simulink model "stepperMotorADRCFirstOrder_originalModel"  (R2026a)
settings: Solver=FixedStepDiscrete  StopTime=1  FixedStep=1e-7
undefined symbols (not defined in the file): alpha_iqd, alpha_s, beta_iqd, beta_s, biq, bs, convert_adc_to_integer, DiscIntNeverNeededParam, electricalRadiansPerCount, gam_iqd, gam_s, k1_iqd, k1_s, KPth, mechanicalRadiansPerCount, PWMVoltage, theta_ref, vs
libraries: simulink x2, mcbeeMathTransformLib x2
settings Model: Creator=mike  LastModifiedBy=drew
settings OptimizationCC: ConditionallyExecuteInputs=off
settings HardwareCC: ProdHWDeviceType=ASIC/FPGA->ASIC/FPGA  TargetBitPerLong=64.0  TargetBitPerPointer=64.0  TargetBitPerSizeT=64.0  TargetBitPerPtrDiffT=64.0  TargetLongLongMode=on  TargetIntDivRoundTo=Zero  TargetEndianess=LittleEndian  TargetWordSize=64.0  TargetHWDeviceType=Custom Processor->MATLAB Host Computer  ProdEqTarget=off

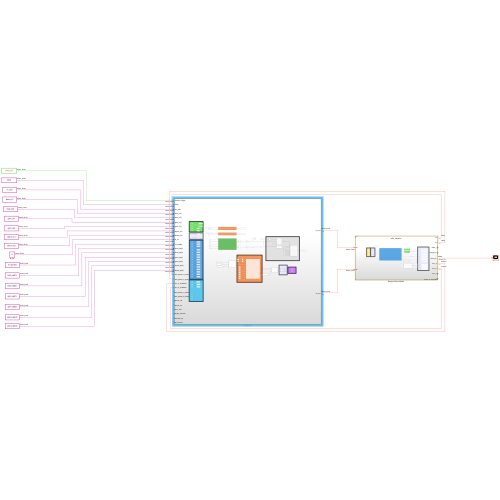
[thumbnail: Simulink's stored preview of the top-level diagram]
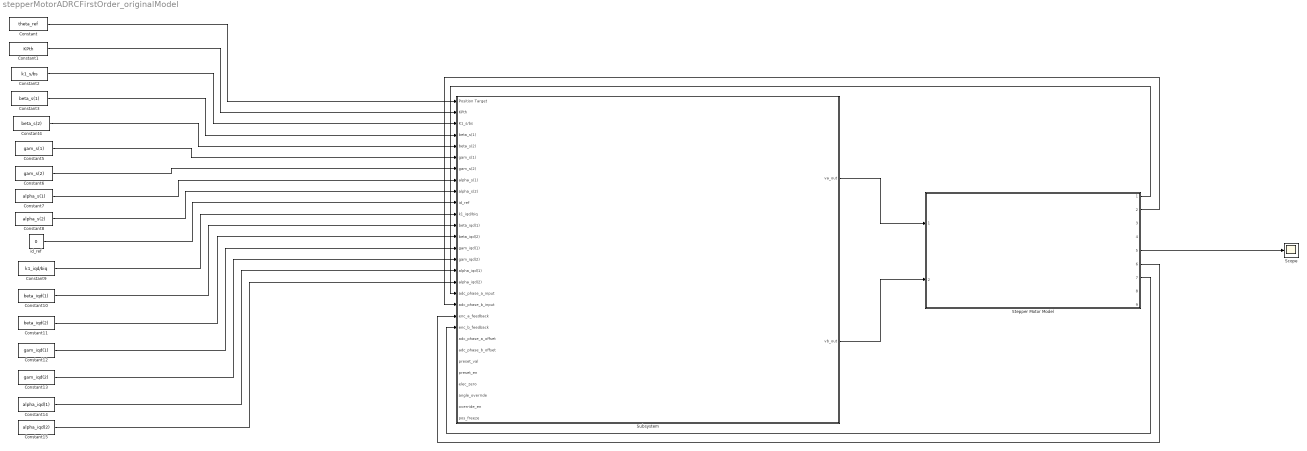
== system stepperMotorADRCFirstOrder_originalModel ==
  Constant : Constant  Value=theta_ref  OutDataTypeStr=PosType  SampleTime=-1
  Constant1 : Constant  Value=KPth  OutDataTypeStr=ParamType
  Constant10 : Constant  Value=beta_iqd(1)  OutDataTypeStr=ParamType
  Constant11 : Constant  Value=beta_iqd(2)  OutDataTypeStr=ParamType
  Constant12 : Constant  Value=gam_iqd(1)  OutDataTypeStr=ParamType
  Constant13 : Constant  Value=gam_iqd(2)  OutDataTypeStr=ParamType
  Constant14 : Constant  Value=alpha_iqd(1)  OutDataTypeStr=ParamType
  Constant15 : Constant  Value=alpha_iqd(2)  OutDataTypeStr=ParamType
  Constant2 : Constant  Value=k1_s/bs  OutDataTypeStr=ParamType
  Constant3 : Constant  Value=beta_s(1)  OutDataTypeStr=ParamType
  Constant4 : Constant  Value=beta_s(2)  OutDataTypeStr=ParamType
  Constant5 : Constant  Value=gam_s(1)  OutDataTypeStr=ParamType
  Constant6 : Constant  Value=gam_s(2)  OutDataTypeStr=ParamType
  Constant7 : Constant  Value=alpha_s(1)  OutDataTypeStr=ParamType
  Constant8 : Constant  Value=alpha_s(2)  OutDataTypeStr=ParamType
  Constant9 : Constant  Value=k1_iqd/biq  OutDataTypeStr=ParamType
  Scope : Scope
      settings: ActiveDisplayYMinimum=-2.1882188276409535  ActiveDisplayYMaximum=0.47029043106523327
  "Stepper Motor Model " : Subsystem  ReferencedSubsystem=adrc_harness
  Subsystem : Subsystem
  id_ref : Constant  Value=0  OutDataTypeStr=ParamType
  wires:
  Constant/1 -> Subsystem/1(Position Target)
  Constant1/1 -> Subsystem/2(KPth)
  Constant2/1 -> Subsystem/3(K1_s/bs)
  Constant3/1 -> Subsystem/4(beta_s(1))
  Constant4/1 -> Subsystem/5(beta_s(2))
  Constant5/1 -> Subsystem/6(gam_s(1))
  Constant6/1 -> Subsystem/7(gam_s(2))
  Constant7/1 -> Subsystem/8(alpha_s(1))
  Constant8/1 -> Subsystem/9(alpha_s(2))
  id_ref/1 -> Subsystem/10(id_ref)
  Constant9/1 -> Subsystem/11(k1_iqd/biq)
  Constant10/1 -> Subsystem/12(beta_iqd(1))
  Constant11/1 -> Subsystem/13(beta_iqd(2))
  Constant12/1 -> Subsystem/14(gam_iqd(1))
  Constant13/1 -> Subsystem/15(gam_iqd(2))
  Constant14/1 -> Subsystem/16(alpha_iqd(1))
  Constant15/1 -> Subsystem/17(alpha_iqd(2))
  Subsystem/1(va_out) -> "Stepper Motor Model "/1
  Subsystem/2(vb_out) -> "Stepper Motor Model "/2
  "Stepper Motor Model "/7 -> Subsystem/21(enc_b_feedback)
  "Stepper Motor Model "/6 -> Subsystem/20(enc_a_feedback)
  "Stepper Motor Model "/1 -> Subsystem/18(adc_phase_a_input)
  "Stepper Motor Model "/2 -> Subsystem/19(adc_phase_b_input)
  "Stepper Motor Model "/5 -> Scope/1

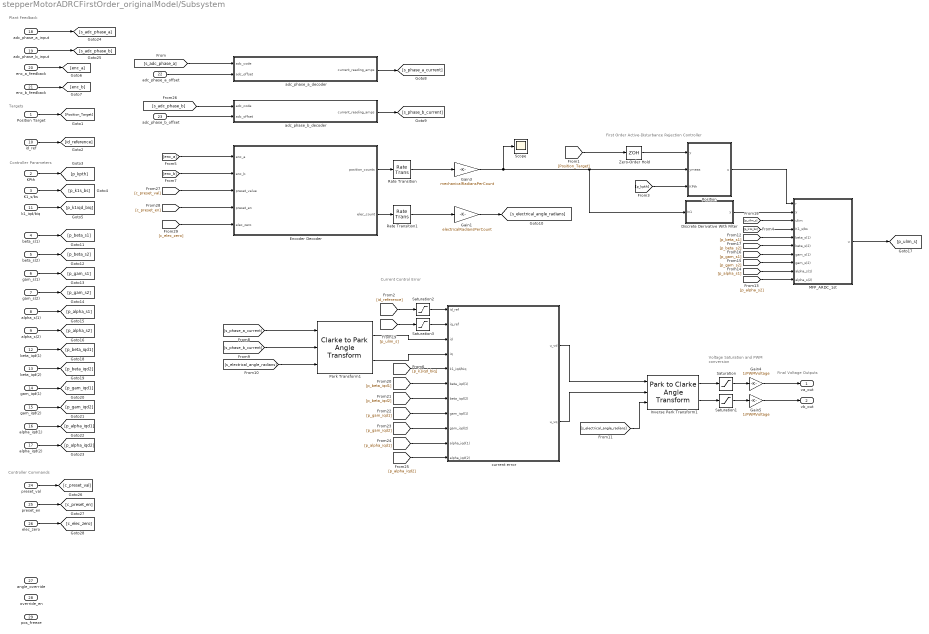
== system stepperMotorADRCFirstOrder_originalModel/Subsystem ==
  note: Final Voltage Outputs
  note: Voltage Saturation and
      | PWM conversion
  note: Current Control Error
  note: First Order Active-Disturbance Rejection Controller
  note: Controller Commands
  note: Controller Parameters
  note: Targets
  note: Plant Feedback
  Position Target : Inport  OutDataTypeStr=PosType
  KPth : Inport  Port=2  OutDataTypeStr=ParamType
  K1_s/bs : Inport  Port=3  OutDataTypeStr=ParamType
  beta_s(1) : Inport  Port=4  OutDataTypeStr=ParamType
  beta_s(2) : Inport  Port=5  OutDataTypeStr=ParamType
  gam_s(1) : Inport  Port=6  OutDataTypeStr=ParamType
  gam_s(2) : Inport  Port=7  OutDataTypeStr=ParamType
  alpha_s(1) : Inport  Port=8  OutDataTypeStr=ParamType
  alpha_s(2) : Inport  Port=9  OutDataTypeStr=ParamType
  id_ref : Inport  Port=10  OutDataTypeStr=ParamType
  k1_iqd/biq : Inport  Port=11  OutDataTypeStr=ParamType
  beta_iqd(1) : Inport  Port=12  OutDataTypeStr=ParamType
  beta_iqd(2) : Inport  Port=13  OutDataTypeStr=ParamType
  gam_iqd(1) : Inport  Port=14  OutDataTypeStr=ParamType
  gam_iqd(2) : Inport  Port=15  OutDataTypeStr=ParamType
  alpha_iqd(1) : Inport  Port=16  OutDataTypeStr=ParamType
  alpha_iqd(2) : Inport  Port=17  OutDataTypeStr=ParamType
  adc_phase_a_input : Inport  Port=18
  adc_phase_b_input : Inport  Port=19
  enc_a_feedback : Inport  Port=20
  enc_b_feedback : Inport  Port=21
  adc_phase_a_offset : Inport  Port=22  OutDataTypeStr=uint16
  adc_phase_b_offset : Inport  Port=23  OutDataTypeStr=uint16
  preset_val : Inport  Port=24  OutDataTypeStr=fixdt(1,32,0)
  preset_en : Inport  Port=25  OutDataTypeStr=boolean
  elec_zero : Inport  Port=26  OutDataTypeStr=boolean
  angle_override : Inport  Port=27  OutDataTypeStr=uint16
  override_en : Inport  Port=28  OutDataTypeStr=boolean
  pos_freeze : Inport  Port=29  OutDataTypeStr=boolean
  Discrete Derivative With Filter : Subsystem
  Encoder Decoder : Subsystem
  Gain1 : Gain  Gain=electricalRadiansPerCount  OutDataTypeStr=PosType  SaturateOnIntegerOverflow=on
  Gain3 : Gain  Gain=mechanicalRadiansPerCount  OutDataTypeStr=PosType  SaturateOnIntegerOverflow=on
  Gain4 : Gain  Gain=1/PWMVoltage  OutDataTypeStr=ParamType
  Gain5 : Gain  Gain=1/PWMVoltage  OutDataTypeStr=ParamType
  Inverse Park Transform1 : mcbeeMathTransformLib/Park to Clarke Angle Transform  AxisAlignment=D-axis  UseWithEmbedded=on  PhaseInput=Two inputs  ThetaInput=Electrical position  AngleInput=Radians  N_points=1024
      settings: LibrarySourceBlock=mcbhdllib/Controls/Math Transforms/Inverse Park Transform
  MFP_ARDC_1st : Subsystem
  Park Transform1 : mcbeeMathTransformLib/Clarke to Park Angle Transform  AxisAlignment=D-axis  UseWithEmbedded=on  PhaseInput=Two inputs  ThetaInput=Electrical position  AngleInput=Radians  N_points=1024
      settings: LibrarySourceBlock=mcbhdllib/Controls/Math Transforms/Park Transform
  "Position " : Subsystem
  Rate Transition : RateTransition  OutPortSampleTime=2e-5
  Rate Transition1 : RateTransition  OutPortSampleTime=2e-5
  Saturation : Saturate  UpperLimit=PWMVoltage  LowerLimit=-PWMVoltage
  Saturation1 : Saturate  UpperLimit=PWMVoltage  LowerLimit=-PWMVoltage  OutDataTypeStr=ParamType
  Saturation2 : Saturate  UpperLimit=2.4  LowerLimit=-2.4  OutDataTypeStr=ParamType
  Saturation3 : Saturate  UpperLimit=2.4  LowerLimit=-2.4  OutDataTypeStr=ParamType
  Scope : Scope
      settings: DataLoggingVariableName=ScopeData3
  Zero-Order Hold : ZeroOrderHold  SampleTime=2e-5
  adc_phase_a_decoder : Subsystem
  adc_phase_b_decoder : Subsystem
  current error : Subsystem
  va_out : Outport  OutDataTypeStr=ParamType
  vb_out : Outport  Port=2  OutDataTypeStr=ParamType
  wires:
  Inverse Park Transform1/2 -> Saturation1/1
  current error/1(u_vd) -> Inverse Park Transform1/1
  current error/2(u_vq) -> Inverse Park Transform1/2
  Zero-Order Hold/1 -> "Position "/1(y)
  Park Transform1/2 -> current error/4(iq)
  Inverse Park Transform1/1 -> Saturation/1
  Park Transform1/1 -> current error/3(id)
  "Position "/1(u) -> MFP_ARDC_1st/1(r)
  Discrete Derivative With Filter/1(y) -> MFP_ARDC_1st/2(y)
  Saturation/1 -> Gain4/1
  Saturation1/1 -> Gain5/1
  Gain4/1 -> va_out/1
  Gain5/1 -> vb_out/1
  [Position_Target] -> Zero-Order Hold/1
  Position Target/1 -> [Position_Target]
  id_ref/1 -> [id_reference]
  [p_kpth] -> "Position "/3(KPth)
  KPth/1 -> [p_kpth]
  [p_k1s_bs] -> MFP_ARDC_1st/4(K1_s/bs)
  K1_s/bs/1 -> [p_k1s_bs]
  [p_k1iqd_biq] -> current error/5(k1_iqd/biq)
  k1_iqd/biq/1 -> [p_k1iqd_biq]
  adc_phase_a_offset/1 -> adc_phase_a_decoder/2(adc_offset)
  adc_phase_b_offset/1 -> adc_phase_b_decoder/2(adc_offset)
  enc_a_feedback/1 -> [enc_a]
  enc_b_feedback/1 -> [enc_b]
  [enc_a] -> Encoder Decoder/1(enc_a)
  [enc_b] -> Encoder Decoder/2(enc_b)
  adc_phase_a_decoder/1(current_reading_amps) -> [s_phase_a_current]
  adc_phase_b_decoder/1(current_reading_amps) -> [s_phase_b_current]
  [s_phase_a_current] -> Park Transform1/1
  [s_phase_b_current] -> Park Transform1/2
  [s_electrical_angle_radians] -> Park Transform1/3
  [s_electrical_angle_radians] -> Inverse Park Transform1/3
  [p_beta_s1] -> MFP_ARDC_1st/5(beta_s(1))
  [p_beta_s2] -> MFP_ARDC_1st/6(beta_s(2))
  [p_gam_s1] -> MFP_ARDC_1st/7(gam_s(1))
  [p_gam_s2] -> MFP_ARDC_1st/8(gam_s(2))
  [p_alpha_s1] -> MFP_ARDC_1st/9(alpha_s(1))
  [p_alpha_s2] -> MFP_ARDC_1st/10(alpha_s(2))
  alpha_s(2)/1 -> [p_alpha_s2]
  alpha_s(1)/1 -> [p_alpha_s1]
  gam_s(2)/1 -> [p_gam_s2]
  gam_s(1)/1 -> [p_gam_s1]
  beta_s(2)/1 -> [p_beta_s2]
  beta_s(1)/1 -> [p_beta_s1]
  MFP_ARDC_1st/1(u) -> [p_ulim_s]
  [p_ulim_s] -> MFP_ARDC_1st/3(ulim)
  beta_iqd(1)/1 -> [p_beta_iqd1]
  beta_iqd(2)/1 -> [p_beta_iqd2]
  [p_beta_iqd2] -> current error/7(beta_iqd(2))
  [p_beta_iqd1] -> current error/6(beta_iqd(1))
  gam_iqd(2)/1 -> [p_gam_iqd2]
  gam_iqd(1)/1 -> [p_gam_iqd1]
  [p_gam_iqd1] -> current error/8(gam_iqd(1))
  [p_gam_iqd2] -> current error/9(gam_iqd(2))
  [p_alpha_iqd1] -> current error/10(alpha_iqd(1))
  [p_alpha_iqd2] -> current error/11(alpha_iqd(2))
  alpha_iqd(1)/1 -> [p_alpha_iqd1]
  alpha_iqd(2)/1 -> [p_alpha_iqd2]
  adc_phase_a_input/1 -> [s_adc_phase_a]
  adc_phase_b_input/1 -> [s_adc_phase_b]
  [s_adc_phase_a] -> adc_phase_a_decoder/1(adc_code)
  [s_adc_phase_b] -> adc_phase_b_decoder/1(adc_code)
  [c_elec_zero] -> Encoder Decoder/5(elec_zero)
  [c_preset_en] -> Encoder Decoder/4(preset_en)
  [c_preset_val] -> Encoder Decoder/3(preset_value)
  elec_zero/1 -> [c_elec_zero]
  preset_en/1 -> [c_preset_en]
  preset_val/1 -> [c_preset_val]
  [id_reference] -> Saturation2/1
  Saturation2/1 -> current error/1(id_ref)
  [p_ulim_s] -> Saturation3/1
  Saturation3/1 -> current error/2(iq_ref)
  Encoder Decoder/2(elec_count) -> Rate Transition1/1
  Encoder Decoder/1(position_counts) -> Rate Transition/1
  Rate Transition/1 -> Gain3/1
  Rate Transition1/1 -> Gain1/1
  Gain1/1 -> [s_electrical_angle_radians]
  Gain3/1 -> Scope/1, Discrete Derivative With Filter/1(In1), "Position "/2(ymeas)

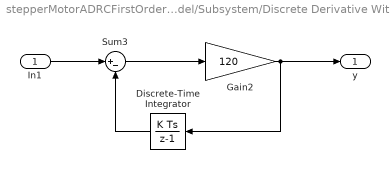
== system stepperMotorADRCFirstOrder_originalModel/Subsystem/Discrete Derivative With Filter ==
  In1 : Inport  OutDataTypeStr=PosType
  Discrete-Time Integrator : DiscreteIntegrator  SampleTime=2e-5  OutDataTypeStr=PosType  SaturateOnIntegerOverflow=on  ICPrevOutput=DiscIntNeverNeededParam  ICPrevScaledInput=DiscIntNeverNeededParam
  Gain2 : Gain  Gain=120  OutDataTypeStr=PosType  ParamDataTypeStr=Inherit: Same as input
  Sum3 : Sum  Inputs=|+-  OutDataTypeStr=PosType
  y : Outport  OutDataTypeStr=PosType
  wires:
  Gain2/1 -> y/1, Discrete-Time Integrator/1
  Sum3/1 -> Gain2/1
  Discrete-Time Integrator/1 -> Sum3/2
  In1/1 -> Sum3/1

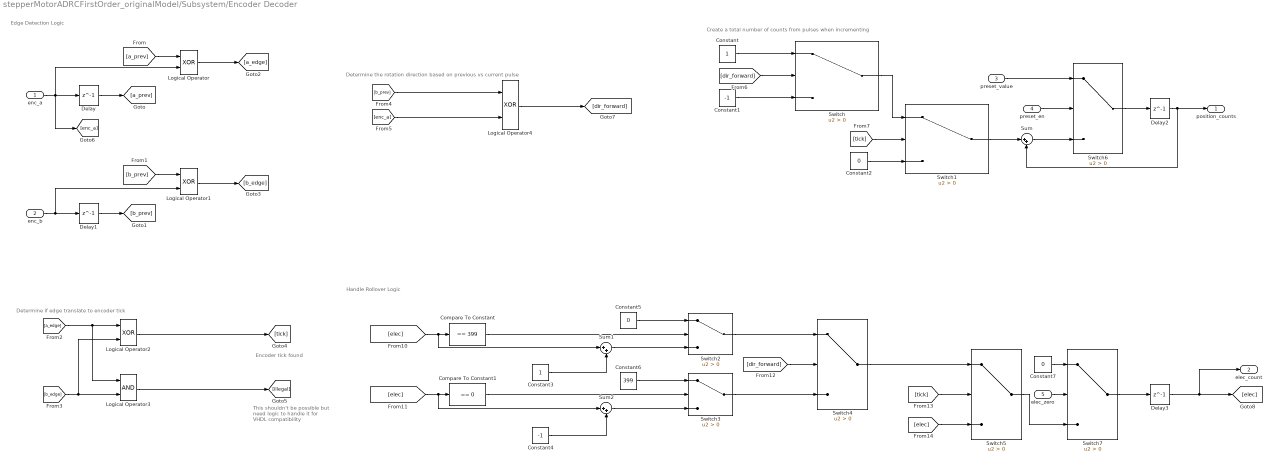
== system stepperMotorADRCFirstOrder_originalModel/Subsystem/Encoder Decoder ==
  note: Handle Rollover Logic
  note: Create a total number of counts from pulses when incrementing
  note: Determine the rotation direction based on previous vs current pulse
  note: Encoder tick found
  note: Determine if edge translate to encoder tick
  note: Edge Detection Logic
  note: This shouldn't be possible but need logic to handle it for VHDL compatibility
  enc_a : Inport  OutDataTypeStr=boolean
  enc_b : Inport  Port=2  OutDataTypeStr=boolean
  preset_value : Inport  Port=3  OutDataTypeStr=fixdt(1,32,0)
  preset_en : Inport  Port=4  OutDataTypeStr=boolean
  elec_zero : Inport  Port=5  OutDataTypeStr=boolean
  Compare To Constant : simulink/Logic and Bit Operations/Compare To Constant  relop===  const=399  OutDataTypeStr=boolean
  Compare To Constant1 : simulink/Logic and Bit Operations/Compare To Constant  relop===  const=0  OutDataTypeStr=boolean
  Constant : Constant  OutDataTypeStr=int32
  Constant1 : Constant  Value=-1  OutDataTypeStr=int32
  Constant2 : Constant  Value=0  OutDataTypeStr=int32
  Constant3 : Constant  OutDataTypeStr=int32
  Constant4 : Constant  Value=-1  OutDataTypeStr=int32
  Constant5 : Constant  Value=0  OutDataTypeStr=int32
  Constant6 : Constant  Value=399  OutDataTypeStr=int32
  Constant7 : Constant  Value=0  OutDataTypeStr=int32
  Delay{,1..3} (4 alike) : Delay  DelayLength=1  InputProcessing=Columns as channels (frame based)  SampleTime=1e-7
  Logical Operator{,1..2,4} (4 alike) : Logic  Operator=XOR  AllPortsSameDT=off  OutDataTypeStr=boolean
  Logical Operator3 : Logic  AllPortsSameDT=off  OutDataTypeStr=boolean
  Sum : Sum  Inputs=|++  OutDataTypeStr=int32  SaturateOnIntegerOverflow=on
  Sum1 : Sum  Inputs=|++  OutDataTypeStr=int32
  Sum2 : Sum  Inputs=|++  OutDataTypeStr=int32
  Switch{,1..5} (6 alike) : Switch  Criteria=u2 > Threshold  SaturateOnIntegerOverflow=off  InputSameDT=off
  Switch6 : Switch  Criteria=u2 > Threshold  OutDataTypeStr=CountType  SaturateOnIntegerOverflow=off  InputSameDT=off
  Switch7 : Switch  Criteria=u2 > Threshold  OutDataTypeStr=CountType  SaturateOnIntegerOverflow=off  InputSameDT=off
  position_counts : Outport  OutDataTypeStr=CountType
  elec_count : Outport  Port=2  OutDataTypeStr=CountType
  wires:
  enc_b/1 -> Logical Operator1/2, Delay1/1
  enc_a/1 -> [enc_a], Logical Operator/2, Delay/1
  Delay/1 -> [a_prev]
  Delay1/1 -> [b_prev]
  [b_prev] -> Logical Operator1/1
  [a_prev] -> Logical Operator/1
  Logical Operator/1 -> [a_edge]
  Logical Operator1/1 -> [b_edge]
  [b_edge] -> Logical Operator3/2, Logical Operator2/2
  [a_edge] -> Logical Operator2/1, Logical Operator3/1
  Logical Operator2/1 -> [tick]
  Logical Operator3/1 -> [illegal]
  [b_prev] -> Logical Operator4/1
  [enc_a] -> Logical Operator4/2
  Logical Operator4/1 -> [dir_forward]
  Constant/1 -> Switch/1
  Constant1/1 -> Switch/3
  [dir_forward] -> Switch/2
  [tick] -> Switch1/2
  Constant2/1 -> Switch1/3
  Switch/1 -> Switch1/1
  Switch1/1 -> Sum/1
  Delay2/1 -> position_counts/1, Sum/2
  Constant5/1 -> Switch2/1
  Compare To Constant1/1 -> Switch3/2
  Sum2/1 -> Switch3/3
  Sum1/1 -> Switch2/3
  Constant6/1 -> Switch3/1
  [elec] -> Sum2/1, Compare To Constant1/1
  [elec] -> Sum1/1, Compare To Constant/1
  Switch2/1 -> Switch4/1
  Constant3/1 -> Sum1/2
  Compare To Constant/1 -> Switch2/2
  Constant4/1 -> Sum2/2
  [dir_forward] -> Switch4/2
  Switch3/1 -> Switch4/3
  Switch4/1 -> Switch5/1
  [tick] -> Switch5/2
  [elec] -> Switch5/3
  Delay3/1 -> elec_count/1, [elec]
  Sum/1 -> Switch6/3
  Switch6/1 -> Delay2/1
  preset_en/1 -> Switch6/2
  preset_value/1 -> Switch6/1
  Constant7/1 -> Switch7/1
  elec_zero/1 -> Switch7/2
  Switch5/1 -> Switch7/3
  Switch7/1 -> Delay3/1

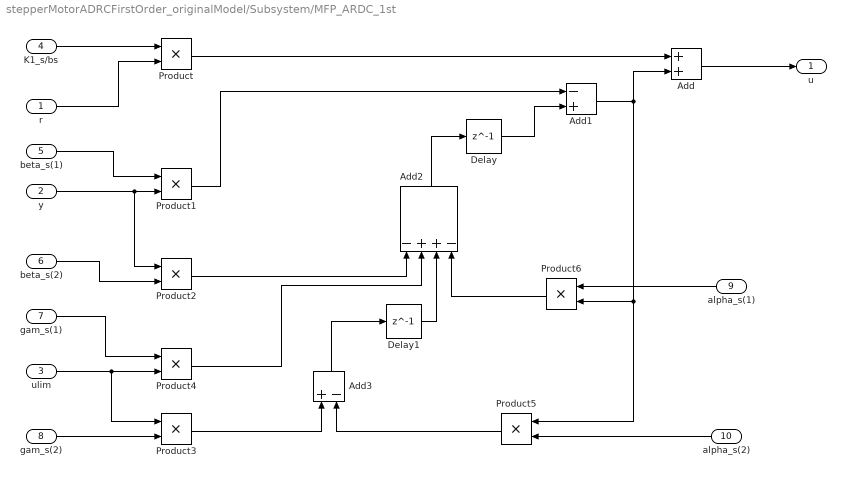
== system stepperMotorADRCFirstOrder_originalModel/Subsystem/MFP_ARDC_1st ==
  r : Inport  OutDataTypeStr=PosType
  y : Inport  Port=2  OutDataTypeStr=PosType
  ulim : Inport  Port=3  OutDataTypeStr=ParamType
  K1_s/bs : Inport  Port=4  OutDataTypeStr=ParamType
  beta_s(1) : Inport  Port=5  OutDataTypeStr=ParamType
  beta_s(2) : Inport  Port=6  OutDataTypeStr=ParamType
  gam_s(1) : Inport  Port=7  OutDataTypeStr=ParamType
  gam_s(2) : Inport  Port=8  OutDataTypeStr=ParamType
  alpha_s(1) : Inport  Port=9  OutDataTypeStr=ParamType
  alpha_s(2) : Inport  Port=10  OutDataTypeStr=ParamType
  Add : Sum  OutDataTypeStr=ParamType  SaturateOnIntegerOverflow=on
  Add1 : Sum  Inputs=-+  OutDataTypeStr=ParamType  SaturateOnIntegerOverflow=on
  Add2 : Sum  Inputs=-++-  OutDataTypeStr=ParamType  SaturateOnIntegerOverflow=on
  Add3 : Sum  Inputs=+-  OutDataTypeStr=ParamType  SaturateOnIntegerOverflow=on
  Delay : Delay  DelayLength=1  InitialCondition=0  SampleTime=2e-5
  Delay1 : Delay  DelayLength=1  InitialCondition=0  SampleTime=2e-5
  Product{,1..6} (7 alike) : Product  OutDataTypeStr=ParamType  SaturateOnIntegerOverflow=on
  u : Outport  OutDataTypeStr=ParamType
  wires:
  Add/1 -> u/1
  Add3/1 -> Delay1/1
  Product4/1 -> Add2/2
  Product6/1 -> Add2/4
  Add1/1 -> Product5/1, Product6/2, Add/2
  Add2/1 -> Delay/1
  r/1 -> Product/2
  Delay1/1 -> Add2/3
  Product3/1 -> Add3/1
  ulim/1 -> Product3/1, Product4/2
  Product2/1 -> Add2/1
  Product5/1 -> Add3/2
  Delay/1 -> Add1/2
  Product1/1 -> Add1/1
  y/1 -> Product2/1, Product1/2
  K1_s/bs/1 -> Product/1
  Product/1 -> Add/1
  beta_s(1)/1 -> Product1/1
  beta_s(2)/1 -> Product2/2
  gam_s(1)/1 -> Product4/1
  gam_s(2)/1 -> Product3/2
  alpha_s(2)/1 -> Product5/2
  alpha_s(1)/1 -> Product6/1

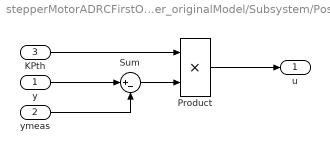
== system stepperMotorADRCFirstOrder_originalModel/Subsystem/Position  ==
  y : Inport  OutDataTypeStr=PosType
  ymeas : Inport  Port=2  OutDataTypeStr=PosType
  KPth : Inport  Port=3  OutDataTypeStr=ParamType
  Product : Product  OutDataTypeStr=PosType  SaturateOnIntegerOverflow=on
  Sum : Sum  Inputs=|+-  OutDataTypeStr=PosType  SaturateOnIntegerOverflow=on
  u : Outport  OutDataTypeStr=PosType
  wires:
  y/1 -> Sum/1
  ymeas/1 -> Sum/2
  Sum/1 -> Product/2
  Product/1 -> u/1
  KPth/1 -> Product/1

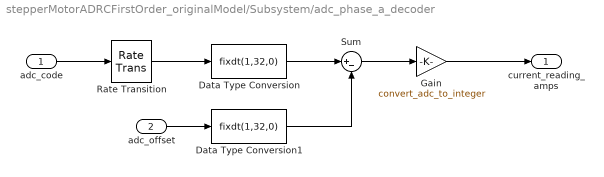
== system stepperMotorADRCFirstOrder_originalModel/Subsystem/adc_phase_a_decoder ==
  adc_code : Inport  OutMin=[0]  OutDataTypeStr=uint16
  adc_offset : Inport  Port=2  OutDataTypeStr=uint16
  Data Type Conversion : DataTypeConversion  OutDataTypeStr=fixdt(1,32,0)  RndMeth=Floor
  Data Type Conversion1 : DataTypeConversion  OutDataTypeStr=fixdt(1,32,0)  RndMeth=Floor
  Gain : Gain  Gain=convert_adc_to_integer  ParamDataTypeStr=fixdt(0,32,38)  OutDataTypeStr=ParamType  RndMeth=Nearest  SaturateOnIntegerOverflow=on
  Rate Transition : RateTransition  OutPortSampleTime=2e-5
  Sum : Sum  Inputs=|+-  OutDataTypeStr=ParamType  AccumDataTypeStr=fixdt(1,32,0)  SaturateOnIntegerOverflow=on
  current_reading_amps : Outport  OutDataTypeStr=ParamType
  wires:
  adc_offset/1 -> Data Type Conversion1/1
  Data Type Conversion1/1 -> Sum/2
  Data Type Conversion/1 -> Sum/1
  Sum/1 -> Gain/1
  Gain/1 -> current_reading_amps/1
  adc_code/1 -> Rate Transition/1
  Rate Transition/1 -> Data Type Conversion/1

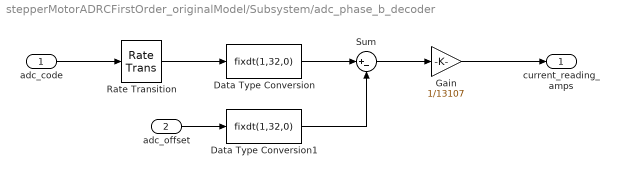
== system stepperMotorADRCFirstOrder_originalModel/Subsystem/adc_phase_b_decoder ==
  adc_code : Inport  OutMin=[0]  OutDataTypeStr=uint16
  adc_offset : Inport  Port=2  OutDataTypeStr=uint16
  Data Type Conversion : DataTypeConversion  OutDataTypeStr=fixdt(1,32,0)  RndMeth=Floor
  Data Type Conversion1 : DataTypeConversion  OutDataTypeStr=fixdt(1,32,0)  RndMeth=Floor
  Gain : Gain  Gain=1/13107  ParamDataTypeStr=fixdt(0,32,38)  OutDataTypeStr=ParamType  RndMeth=Nearest  SaturateOnIntegerOverflow=on
  Rate Transition : RateTransition  OutPortSampleTime=2e-5
  Sum : Sum  Inputs=|+-  OutDataTypeStr=ParamType  AccumDataTypeStr=fixdt(1,32,0)  SaturateOnIntegerOverflow=on
  current_reading_amps : Outport  OutDataTypeStr=ParamType
  wires:
  adc_offset/1 -> Data Type Conversion1/1
  Data Type Conversion1/1 -> Sum/2
  Data Type Conversion/1 -> Sum/1
  Sum/1 -> Gain/1
  Gain/1 -> current_reading_amps/1
  Rate Transition/1 -> Data Type Conversion/1
  adc_code/1 -> Rate Transition/1

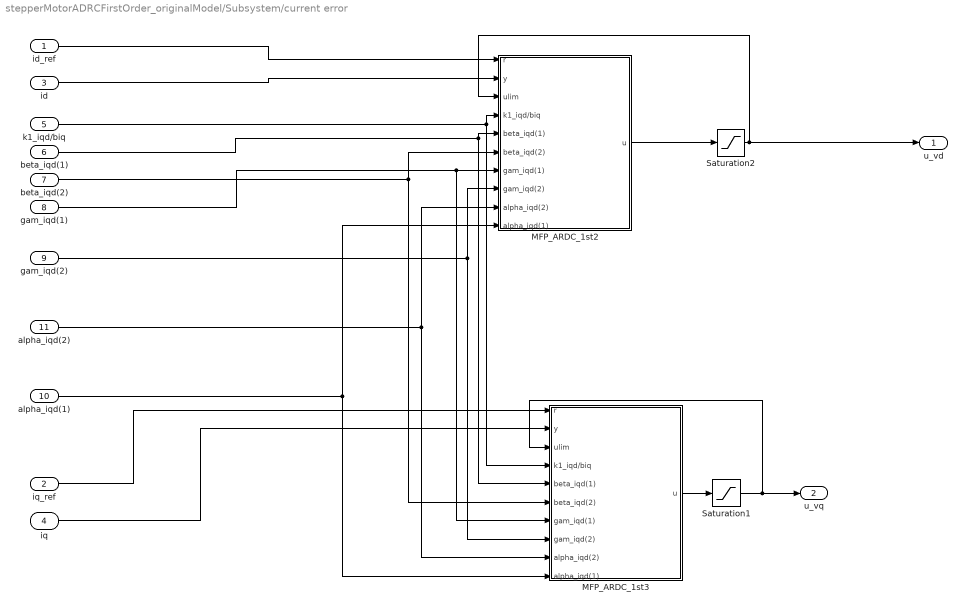
== system stepperMotorADRCFirstOrder_originalModel/Subsystem/current error ==
  id_ref : Inport  OutDataTypeStr=ParamType
  iq_ref : Inport  Port=2  OutDataTypeStr=ParamType
  id : Inport  Port=3  OutDataTypeStr=ParamType
  iq : Inport  Port=4  OutDataTypeStr=ParamType
  k1_iqd/biq : Inport  Port=5  OutDataTypeStr=ParamType
  beta_iqd(1) : Inport  Port=6  OutDataTypeStr=ParamType
  beta_iqd(2) : Inport  Port=7  OutDataTypeStr=ParamType
  gam_iqd(1) : Inport  Port=8  OutDataTypeStr=ParamType
  gam_iqd(2) : Inport  Port=9  OutDataTypeStr=ParamType
  alpha_iqd(1) : Inport  Port=10  OutDataTypeStr=ParamType
  alpha_iqd(2) : Inport  Port=11  OutDataTypeStr=ParamType
  MFP_ARDC_1st2 : Subsystem
  MFP_ARDC_1st3 : Subsystem
  Saturation1 : Saturate  UpperLimit=vs  LowerLimit=-vs  OutDataTypeStr=ParamType
  Saturation2 : Saturate  UpperLimit=vs  LowerLimit=-vs  OutDataTypeStr=ParamType
  u_vd : Outport  OutDataTypeStr=ParamType
  u_vq : Outport  Port=2  OutDataTypeStr=ParamType
  wires:
  iq_ref/1 -> MFP_ARDC_1st3/1(r)
  iq/1 -> MFP_ARDC_1st3/2(y)
  Saturation1/1 -> MFP_ARDC_1st3/3(ulim), u_vq/1
  MFP_ARDC_1st3/1(u) -> Saturation1/1
  id/1 -> MFP_ARDC_1st2/2(y)
  id_ref/1 -> MFP_ARDC_1st2/1(r)
  MFP_ARDC_1st2/1(u) -> Saturation2/1
  Saturation2/1 -> MFP_ARDC_1st2/3(ulim), u_vd/1
  k1_iqd/biq/1 -> MFP_ARDC_1st2/4(k1_iqd/biq), MFP_ARDC_1st3/4(k1_iqd/biq)
  beta_iqd(1)/1 -> MFP_ARDC_1st2/5(beta_iqd(1)), MFP_ARDC_1st3/5(beta_iqd(1))
  beta_iqd(2)/1 -> MFP_ARDC_1st3/6(beta_iqd(2)), MFP_ARDC_1st2/6(beta_iqd(2))
  gam_iqd(1)/1 -> MFP_ARDC_1st2/7(gam_iqd(1)), MFP_ARDC_1st3/7(gam_iqd(1))
  gam_iqd(2)/1 -> MFP_ARDC_1st2/8(gam_iqd(2)), MFP_ARDC_1st3/8(gam_iqd(2))
  alpha_iqd(2)/1 -> MFP_ARDC_1st2/9(alpha_iqd(2)), MFP_ARDC_1st3/9(alpha_iqd(2))
  alpha_iqd(1)/1 -> MFP_ARDC_1st2/10(alpha_iqd(1)), MFP_ARDC_1st3/10(alpha_iqd(1))

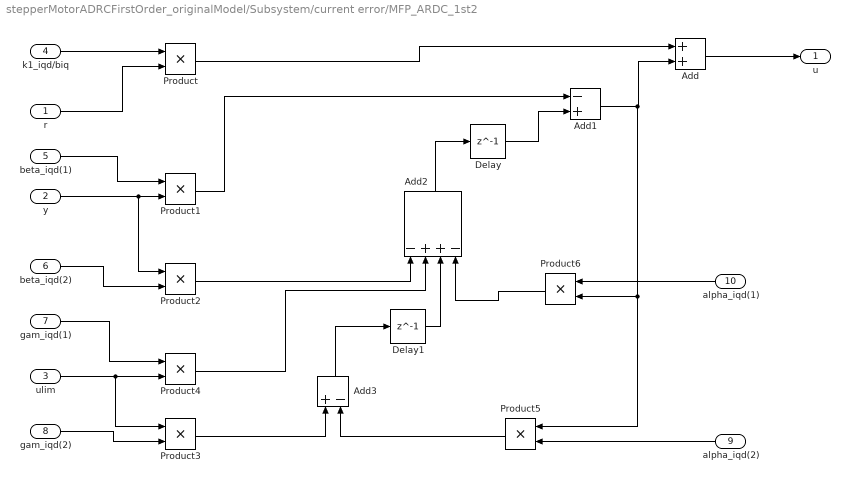
== system stepperMotorADRCFirstOrder_originalModel/Subsystem/current error/MFP_ARDC_1st2 ==
  r : Inport
  y : Inport  Port=2
  ulim : Inport  Port=3
  k1_iqd/biq : Inport  Port=4
  beta_iqd(1) : Inport  Port=5
  beta_iqd(2) : Inport  Port=6
  gam_iqd(1) : Inport  Port=7
  gam_iqd(2) : Inport  Port=8
  alpha_iqd(2) : Inport  Port=9
  alpha_iqd(1) : Inport  Port=10
  Add : Sum  SaturateOnIntegerOverflow=on  OutDataTypeStr=Inherit: Same as first input
  Add1 : Sum  Inputs=-+  SaturateOnIntegerOverflow=on  OutDataTypeStr=Inherit: Same as first input
  Add2 : Sum  Inputs=-++-
  Add3 : Sum  Inputs=+-  SaturateOnIntegerOverflow=on  OutDataTypeStr=Inherit: Same as first input
  Delay : Delay  DelayLength=1  InitialCondition=0  SampleTime=2e-5
  Delay1 : Delay  DelayLength=1  InitialCondition=0  SampleTime=2e-5
  Product{,1..6} (7 alike) : Product  SaturateOnIntegerOverflow=on  OutDataTypeStr=Inherit: Same as first input
  u : Outport
  wires:
  Add/1 -> u/1
  Add3/1 -> Delay1/1
  Product4/1 -> Add2/2
  Product6/1 -> Add2/4
  Add1/1 -> Product5/1, Product6/2, Add/2
  Add2/1 -> Delay/1
  r/1 -> Product/2
  Delay1/1 -> Add2/3
  Product3/1 -> Add3/1
  ulim/1 -> Product3/1, Product4/2
  Product2/1 -> Add2/1
  Product5/1 -> Add3/2
  Delay/1 -> Add1/2
  Product1/1 -> Add1/1
  y/1 -> Product2/1, Product1/2
  k1_iqd/biq/1 -> Product/1
  Product/1 -> Add/1
  beta_iqd(1)/1 -> Product1/1
  beta_iqd(2)/1 -> Product2/2
  gam_iqd(1)/1 -> Product4/1
  gam_iqd(2)/1 -> Product3/2
  alpha_iqd(2)/1 -> Product5/2
  alpha_iqd(1)/1 -> Product6/1

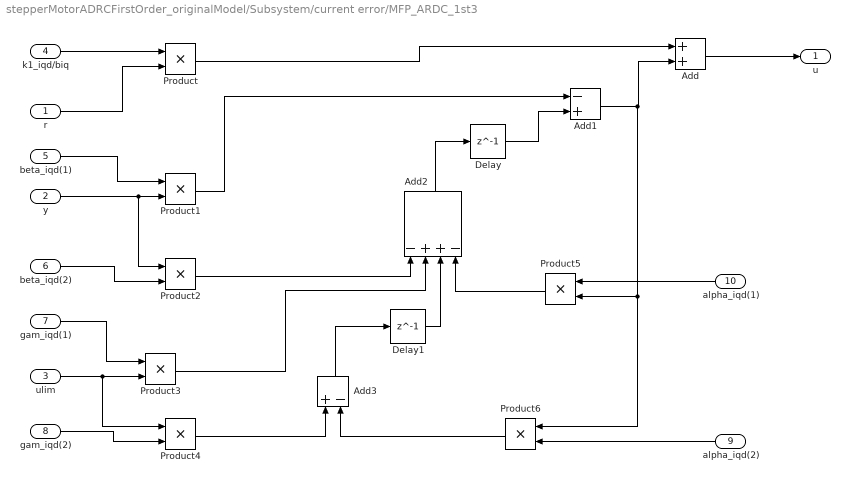
== system stepperMotorADRCFirstOrder_originalModel/Subsystem/current error/MFP_ARDC_1st3 ==
  r : Inport
  y : Inport  Port=2
  ulim : Inport  Port=3
  k1_iqd/biq : Inport  Port=4
  beta_iqd(1) : Inport  Port=5
  beta_iqd(2) : Inport  Port=6
  gam_iqd(1) : Inport  Port=7
  gam_iqd(2) : Inport  Port=8
  alpha_iqd(2) : Inport  Port=9
  alpha_iqd(1) : Inport  Port=10
  Add : Sum  SaturateOnIntegerOverflow=on  OutDataTypeStr=Inherit: Same as first input
  Add1 : Sum  Inputs=-+  SaturateOnIntegerOverflow=on  OutDataTypeStr=Inherit: Same as first input
  Add2 : Sum  Inputs=-++-  SaturateOnIntegerOverflow=on
  Add3 : Sum  Inputs=+-  SaturateOnIntegerOverflow=on  OutDataTypeStr=Inherit: Same as first input
  Delay : Delay  DelayLength=1  InitialCondition=0  SampleTime=2e-5
  Delay1 : Delay  DelayLength=1  InitialCondition=0  SampleTime=2e-5
  Product{,1..6} (7 alike) : Product  SaturateOnIntegerOverflow=on  OutDataTypeStr=Inherit: Same as first input
  u : Outport
  wires:
  Add/1 -> u/1
  Add3/1 -> Delay1/1
  Product3/1 -> Add2/2
  Product5/1 -> Add2/4
  Add1/1 -> Product6/1, Product5/2, Add/2
  Add2/1 -> Delay/1
  r/1 -> Product/2
  Delay1/1 -> Add2/3
  Product4/1 -> Add3/1
  ulim/1 -> Product4/1, Product3/2
  Product2/1 -> Add2/1
  Product6/1 -> Add3/2
  Delay/1 -> Add1/2
  Product1/1 -> Add1/1
  y/1 -> Product2/1, Product1/2
  k1_iqd/biq/1 -> Product/1
  Product/1 -> Add/1
  beta_iqd(1)/1 -> Product1/1
  beta_iqd(2)/1 -> Product2/2
  gam_iqd(1)/1 -> Product3/1
  gam_iqd(2)/1 -> Product4/2
  alpha_iqd(2)/1 -> Product6/2
  alpha_iqd(1)/1 -> Product5/1
